simulink model "P1"  (R2017b)
settings: Solver=VariableStepAuto  StartTime=0.0  StopTime=20  RelTol=1e-3
settings Model: Creator=Cx001la  LastModifiedBy=Cx001la

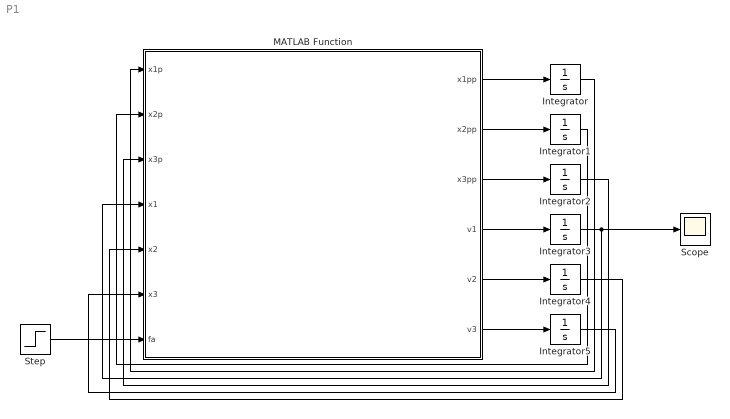
== system P1 ==
  Integrator{,1..5} (6 alike) : Integrator
  MATLAB Function : MATLAB Function  TreatAsAtomicUnit=on
  Scope : Scope
  Step : Step  Time=0  SampleTime=0
  wires:
  MATLAB Function/1(x1pp) -> Integrator/1
  MATLAB Function/2(x2pp) -> Integrator1/1
  MATLAB Function/3(x3pp) -> Integrator2/1
  MATLAB Function/4(v1) -> Integrator3/1
  MATLAB Function/5(v2) -> Integrator4/1
  MATLAB Function/6(v3) -> Integrator5/1
  Integrator/1 -> MATLAB Function/1(x1p)
  Integrator1/1 -> MATLAB Function/2(x2p)
  Integrator2/1 -> MATLAB Function/3(x3p)
  Integrator3/1 -> Scope/1, MATLAB Function/4(x1)
  Integrator4/1 -> MATLAB Function/5(x2)
  Integrator5/1 -> MATLAB Function/6(x3)
  Step/1 -> MATLAB Function/7(fa)

== matlab function P1/MATLAB Function ==
  data: x1p input; x1pp output; x2p input; x3p input; x1 input; x2 input; x3 input; fa input; x2pp output; x3pp output; v1 output; v2 output; v3 output
function [x1pp,x2pp,x3pp,v1,v2,v3] = fcn( x1p,x2p,x3p,x1,x2,x3,fa)
m1=0.2; m2=0.5; m3=0.3; g=9.81; k1=100; k2=150; k3=50; k4=110; b1=20; b2=50;

x1pp=(  -k1*(x1-x2)-2*b1*(x1p-x3p)+m1*g  )/(m1);
x2pp= (  -2*b2*(x2p-x3p)-k2*(x2-x3)+k1*(x1-x2)+m2*g  )/(m2);
x3pp=(  2*b1*(x1p-x3p)+2*b2*(x2p-x3p)+k2*(x1-x3)-0.7*k4*x3-0.7*k3*x3-fa  )/(m3);
v1=x1p;
v2=x2p;
v3=x3p;
